simulink library "VIS_LIB"  (Simulink 8.6)
settings: Solver=ode45  StartTime=0.0  StopTime=10.0  RelTol=1e-3
undefined symbols (not defined in the file): AC, SIXOSEM_F_WD_AC_MASTER
libraries: cdsFilt x376, cdsEpicsOut x253, cdsEpicsIn x179, cdsTP x123, VIS_LIB x95, cdsMuxMatrix x91, cdsEpicsStringIn x75, cdsFiltCtrl x72, cdsFunctionCall x70, cdsRms x59, KAGRA_UTIL x25, STATE_BIO_MASTER x5
(part 19 of 38)

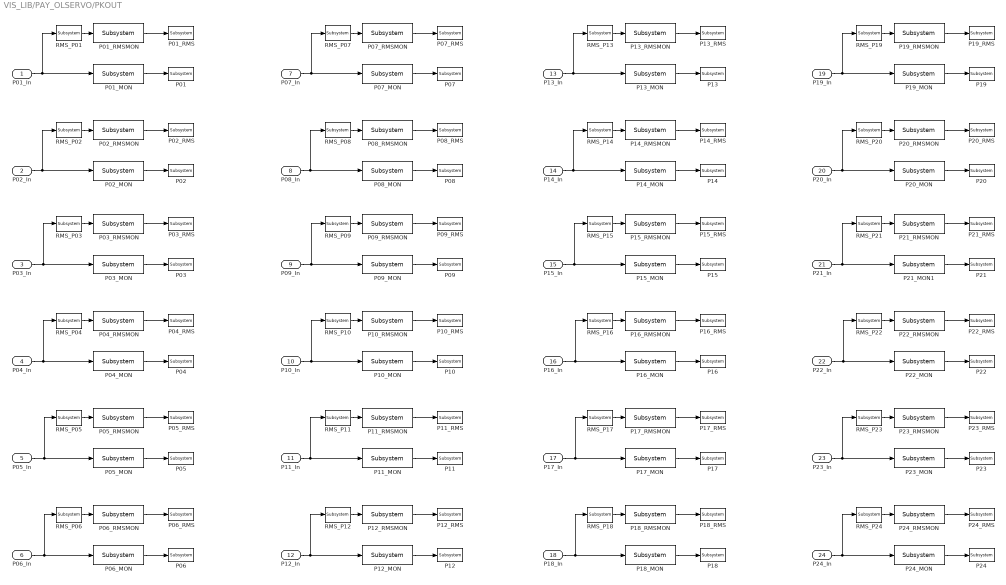
== system VIS_LIB/PAY_OLSERVO/PKOUT ==
  P01_In : Inport
  P02_In : Inport  Port=2
  P03_In : Inport  Port=3
  P04_In : Inport  Port=4
  P05_In : Inport  Port=5
  P06_In : Inport  Port=6
  P07_In : Inport  Port=7
  P08_In : Inport  Port=8
  P09_In : Inport  Port=9
  P10_In : Inport  Port=10
  P11_In : Inport  Port=11
  P12_In : Inport  Port=12
  P13_In : Inport  Port=13
  P14_In : Inport  Port=14
  P15_In : Inport  Port=15
  P16_In : Inport  Port=16
  P17_In : Inport  Port=17
  P18_In : Inport  Port=18
  P19_In : Inport  Port=19
  P20_In : Inport  Port=20
  P21_In : Inport  Port=21
  P22_In : Inport  Port=22
  P23_In : Inport  Port=23
  P24_In : Inport  Port=24
  P01 : cdsTP/Subsystem  Tag=Test Point
      settings: AttributesFormatString=%<Tag>
  P01_MON : cdsEpicsOut/Subsystem  Tag=cdsEpicsOutput  Description=|
      | Purpose:                                          
      | Output a FE signal to an EPICS channel.           
      |                                                   
      | Operation:                                        
      | Takes input value and passes it to EPICS record.  
      |                                                   
      | Usage:                                            
      | Name the part with the desired EPICS rrecord name.
      settings: AttributesFormatString=%<Tag>
  P01_RMS : cdsTP/Subsystem  Tag=Test Point
      settings: AttributesFormatString=%<Tag>
  P01_RMSMON : cdsEpicsOut/Subsystem  Tag=cdsEpicsOutput  Description=|
      | Purpose:                                          
      | Output a FE signal to an EPICS channel.           
      |                                                   
      | Operation:                                        
      | Takes input value and passes it to EPICS record.  
      |                                                   
      | Usage:                                            
      | Name the part with the desired EPICS rrecord name.
      settings: AttributesFormatString=%<Tag>
  P02 : cdsTP/Subsystem  Tag=Test Point
      settings: AttributesFormatString=%<Tag>
  P02_MON : cdsEpicsOut/Subsystem  Tag=cdsEpicsOutput  Description=|
      | Purpose:                                          
      | Output a FE signal to an EPICS channel.           
      |                                                   
      | Operation:                                        
      | Takes input value and passes it to EPICS record.  
      |                                                   
      | Usage:                                            
      | Name the part with the desired EPICS rrecord name.
      settings: AttributesFormatString=%<Tag>
  P02_RMS : cdsTP/Subsystem  Tag=Test Point
      settings: AttributesFormatString=%<Tag>
  P02_RMSMON : cdsEpicsOut/Subsystem  Tag=cdsEpicsOutput  Description=|
      | Purpose:                                          
      | Output a FE signal to an EPICS channel.           
      |                                                   
      | Operation:                                        
      | Takes input value and passes it to EPICS record.  
      |                                                   
      | Usage:                                            
      | Name the part with the desired EPICS rrecord name.
      settings: AttributesFormatString=%<Tag>
  P03 : cdsTP/Subsystem  Tag=Test Point
      settings: AttributesFormatString=%<Tag>
  P03_MON : cdsEpicsOut/Subsystem  Tag=cdsEpicsOutput  Description=|
      | Purpose:                                          
      | Output a FE signal to an EPICS channel.           
      |                                                   
      | Operation:                                        
      | Takes input value and passes it to EPICS record.  
      |                                                   
      | Usage:                                            
      | Name the part with the desired EPICS rrecord name.
      settings: AttributesFormatString=%<Tag>
  P03_RMS : cdsTP/Subsystem  Tag=Test Point
      settings: AttributesFormatString=%<Tag>
  P03_RMSMON : cdsEpicsOut/Subsystem  Tag=cdsEpicsOutput  Description=|
      | Purpose:                                          
      | Output a FE signal to an EPICS channel.           
      |                                                   
      | Operation:                                        
      | Takes input value and passes it to EPICS record.  
      |                                                   
      | Usage:                                            
      | Name the part with the desired EPICS rrecord name.
      settings: AttributesFormatString=%<Tag>
  P04 : cdsTP/Subsystem  Tag=Test Point
      settings: AttributesFormatString=%<Tag>
  P04_MON : cdsEpicsOut/Subsystem  Tag=cdsEpicsOutput  Description=|
      | Purpose:                                          
      | Output a FE signal to an EPICS channel.           
      |                                                   
      | Operation:                                        
      | Takes input value and passes it to EPICS record.  
      |                                                   
      | Usage:                                            
      | Name the part with the desired EPICS rrecord name.
      settings: AttributesFormatString=%<Tag>
  P04_RMS : cdsTP/Subsystem  Tag=Test Point
      settings: AttributesFormatString=%<Tag>
  P04_RMSMON : cdsEpicsOut/Subsystem  Tag=cdsEpicsOutput  Description=|
      | Purpose:                                          
      | Output a FE signal to an EPICS channel.           
      |                                                   
      | Operation:                                        
      | Takes input value and passes it to EPICS record.  
      |                                                   
      | Usage:                                            
      | Name the part with the desired EPICS rrecord name.
      settings: AttributesFormatString=%<Tag>
  P05 : cdsTP/Subsystem  Tag=Test Point
      settings: AttributesFormatString=%<Tag>
  P05_MON : cdsEpicsOut/Subsystem  Tag=cdsEpicsOutput  Description=|
      | Purpose:                                          
      | Output a FE signal to an EPICS channel.           
      |                                                   
      | Operation:                                        
      | Takes input value and passes it to EPICS record.  
      |                                                   
      | Usage:                                            
      | Name the part with the desired EPICS rrecord name.
      settings: AttributesFormatString=%<Tag>
  P05_RMS : cdsTP/Subsystem  Tag=Test Point
      settings: AttributesFormatString=%<Tag>
  P05_RMSMON : cdsEpicsOut/Subsystem  Tag=cdsEpicsOutput  Description=|
      | Purpose:                                          
      | Output a FE signal to an EPICS channel.           
      |                                                   
      | Operation:                                        
      | Takes input value and passes it to EPICS record.  
      |                                                   
      | Usage:                                            
      | Name the part with the desired EPICS rrecord name.
      settings: AttributesFormatString=%<Tag>
  P06 : cdsTP/Subsystem  Tag=Test Point
      settings: AttributesFormatString=%<Tag>
  P06_MON : cdsEpicsOut/Subsystem  Tag=cdsEpicsOutput  Description=|
      | Purpose:                                          
      | Output a FE signal to an EPICS channel.           
      |                                                   
      | Operation:                                        
      | Takes input value and passes it to EPICS record.  
      |                                                   
      | Usage:                                            
      | Name the part with the desired EPICS rrecord name.
      settings: AttributesFormatString=%<Tag>
  P06_RMS : cdsTP/Subsystem  Tag=Test Point
      settings: AttributesFormatString=%<Tag>
  P06_RMSMON : cdsEpicsOut/Subsystem  Tag=cdsEpicsOutput  Description=|
      | Purpose:                                          
      | Output a FE signal to an EPICS channel.           
      |                                                   
      | Operation:                                        
      | Takes input value and passes it to EPICS record.  
      |                                                   
      | Usage:                                            
      | Name the part with the desired EPICS rrecord name.
      settings: AttributesFormatString=%<Tag>
  P07 : cdsTP/Subsystem  Tag=Test Point
      settings: AttributesFormatString=%<Tag>
  P07_MON : cdsEpicsOut/Subsystem  Tag=cdsEpicsOutput  Description=|
      | Purpose:                                          
      | Output a FE signal to an EPICS channel.           
      |                                                   
      | Operation:                                        
      | Takes input value and passes it to EPICS record.  
      |                                                   
      | Usage:                                            
      | Name the part with the desired EPICS rrecord name.
      settings: AttributesFormatString=%<Tag>
  P07_RMS : cdsTP/Subsystem  Tag=Test Point
      settings: AttributesFormatString=%<Tag>
  P07_RMSMON : cdsEpicsOut/Subsystem  Tag=cdsEpicsOutput  Description=|
      | Purpose:                                          
      | Output a FE signal to an EPICS channel.           
      |                                                   
      | Operation:                                        
      | Takes input value and passes it to EPICS record.  
      |                                                   
      | Usage:                                            
      | Name the part with the desired EPICS rrecord name.
      settings: AttributesFormatString=%<Tag>
  P08 : cdsTP/Subsystem  Tag=Test Point
      settings: AttributesFormatString=%<Tag>
  P08_MON : cdsEpicsOut/Subsystem  Tag=cdsEpicsOutput  Description=|
      | Purpose:                                          
      | Output a FE signal to an EPICS channel.           
      |                                                   
      | Operation:                                        
      | Takes input value and passes it to EPICS record.  
      |                                                   
      | Usage:                                            
      | Name the part with the desired EPICS rrecord name.
      settings: AttributesFormatString=%<Tag>
  P08_RMS : cdsTP/Subsystem  Tag=Test Point
      settings: AttributesFormatString=%<Tag>
  P08_RMSMON : cdsEpicsOut/Subsystem  Tag=cdsEpicsOutput  Description=|
      | Purpose:                                          
      | Output a FE signal to an EPICS channel.           
      |                                                   
      | Operation:                                        
      | Takes input value and passes it to EPICS record.  
      |                                                   
      | Usage:                                            
      | Name the part with the desired EPICS rrecord name.
      settings: AttributesFormatString=%<Tag>
  P09 : cdsTP/Subsystem  Tag=Test Point
      settings: AttributesFormatString=%<Tag>
  P09_MON : cdsEpicsOut/Subsystem  Tag=cdsEpicsOutput  Description=|
      | Purpose:                                          
      | Output a FE signal to an EPICS channel.           
      |                                                   
      | Operation:                                        
      | Takes input value and passes it to EPICS record.  
      |                                                   
      | Usage:                                            
      | Name the part with the desired EPICS rrecord name.
      settings: AttributesFormatString=%<Tag>
  P09_RMS : cdsTP/Subsystem  Tag=Test Point
      settings: AttributesFormatString=%<Tag>
  P09_RMSMON : cdsEpicsOut/Subsystem  Tag=cdsEpicsOutput  Description=|
      | Purpose:                                          
      | Output a FE signal to an EPICS channel.           
      |                                                   
      | Operation:                                        
      | Takes input value and passes it to EPICS record.  
      |                                                   
      | Usage:                                            
      | Name the part with the desired EPICS rrecord name.
      settings: AttributesFormatString=%<Tag>
  P{10..24} (15 alike) : cdsTP/Subsystem  Tag=Test Point
      settings: AttributesFormatString=%<Tag>
  P10_MON : cdsEpicsOut/Subsystem  Tag=cdsEpicsOutput  Description=|
      | Purpose:                                          
      | Output a FE signal to an EPICS channel.           
      |                                                   
      | Operation:                                        
      | Takes input value and passes it to EPICS record.  
      |                                                   
      | Usage:                                            
      | Name the part with the desired EPICS rrecord name.
      settings: AttributesFormatString=%<Tag>
  P10_RMS : cdsTP/Subsystem  Tag=Test Point
      settings: AttributesFormatString=%<Tag>
  P10_RMSMON : cdsEpicsOut/Subsystem  Tag=cdsEpicsOutput  Description=|
      | Purpose:                                          
      | Output a FE signal to an EPICS channel.           
      |                                                   
      | Operation:                                        
      | Takes input value and passes it to EPICS record.  
      |                                                   
      | Usage:                                            
      | Name the part with the desired EPICS rrecord name.
      settings: AttributesFormatString=%<Tag>
  P11_MON : cdsEpicsOut/Subsystem  Tag=cdsEpicsOutput  Description=|
      | Purpose:                                          
      | Output a FE signal to an EPICS channel.           
      |                                                   
      | Operation:                                        
      | Takes input value and passes it to EPICS record.  
      |                                                   
      | Usage:                                            
      | Name the part with the desired EPICS rrecord name.
      settings: AttributesFormatString=%<Tag>
  P11_RMS : cdsTP/Subsystem  Tag=Test Point
      settings: AttributesFormatString=%<Tag>
  P11_RMSMON : cdsEpicsOut/Subsystem  Tag=cdsEpicsOutput  Description=|
      | Purpose:                                          
      | Output a FE signal to an EPICS channel.           
      |                                                   
      | Operation:                                        
      | Takes input value and passes it to EPICS record.  
      |                                                   
      | Usage:                                            
      | Name the part with the desired EPICS rrecord name.
      settings: AttributesFormatString=%<Tag>
  P12_MON : cdsEpicsOut/Subsystem  Tag=cdsEpicsOutput  Description=|
      | Purpose:                                          
      | Output a FE signal to an EPICS channel.           
      |                                                   
      | Operation:                                        
      | Takes input value and passes it to EPICS record.  
      |                                                   
      | Usage:                                            
      | Name the part with the desired EPICS rrecord name.
      settings: AttributesFormatString=%<Tag>
  P12_RMS : cdsTP/Subsystem  Tag=Test Point
      settings: AttributesFormatString=%<Tag>
  P12_RMSMON : cdsEpicsOut/Subsystem  Tag=cdsEpicsOutput  Description=|
      | Purpose:                                          
      | Output a FE signal to an EPICS channel.           
      |                                                   
      | Operation:                                        
      | Takes input value and passes it to EPICS record.  
      |                                                   
      | Usage:                                            
      | Name the part with the desired EPICS rrecord name.
      settings: AttributesFormatString=%<Tag>
  P13_MON : cdsEpicsOut/Subsystem  Tag=cdsEpicsOutput  Description=|
      | Purpose:                                          
      | Output a FE signal to an EPICS channel.           
      |                                                   
      | Operation:                                        
      | Takes input value and passes it to EPICS record.  
      |                                                   
      | Usage:                                            
      | Name the part with the desired EPICS rrecord name.
      settings: AttributesFormatString=%<Tag>
  P13_RMS : cdsTP/Subsystem  Tag=Test Point
      settings: AttributesFormatString=%<Tag>
  P13_RMSMON : cdsEpicsOut/Subsystem  Tag=cdsEpicsOutput  Description=|
      | Purpose:                                          
      | Output a FE signal to an EPICS channel.           
      |                                                   
      | Operation:                                        
      | Takes input value and passes it to EPICS record.  
      |                                                   
      | Usage:                                            
      | Name the part with the desired EPICS rrecord name.
      settings: AttributesFormatString=%<Tag>
  P14_MON : cdsEpicsOut/Subsystem  Tag=cdsEpicsOutput  Description=|
      | Purpose:                                          
      | Output a FE signal to an EPICS channel.           
      |                                                   
      | Operation:                                        
      | Takes input value and passes it to EPICS record.  
      |                                                   
      | Usage:                                            
      | Name the part with the desired EPICS rrecord name.
      settings: AttributesFormatString=%<Tag>
  P14_RMS : cdsTP/Subsystem  Tag=Test Point
      settings: AttributesFormatString=%<Tag>
  P14_RMSMON : cdsEpicsOut/Subsystem  Tag=cdsEpicsOutput  Description=|
      | Purpose:                                          
      | Output a FE signal to an EPICS channel.           
      |                                                   
      | Operation:                                        
      | Takes input value and passes it to EPICS record.  
      |                                                   
      | Usage:                                            
      | Name the part with the desired EPICS rrecord name.
      settings: AttributesFormatString=%<Tag>
  P15_MON : cdsEpicsOut/Subsystem  Tag=cdsEpicsOutput  Description=|
      | Purpose:                                          
      | Output a FE signal to an EPICS channel.           
      |                                                   
      | Operation:                                        
      | Takes input value and passes it to EPICS record.  
      |                                                   
      | Usage:                                            
      | Name the part with the desired EPICS rrecord name.
      settings: AttributesFormatString=%<Tag>
  P15_RMS : cdsTP/Subsystem  Tag=Test Point
      settings: AttributesFormatString=%<Tag>
  P15_RMSMON : cdsEpicsOut/Subsystem  Tag=cdsEpicsOutput  Description=|
      | Purpose:                                          
      | Output a FE signal to an EPICS channel.           
      |                                                   
      | Operation:                                        
      | Takes input value and passes it to EPICS record.  
      |                                                   
      | Usage:                                            
      | Name the part with the desired EPICS rrecord name.
      settings: AttributesFormatString=%<Tag>
  P16_MON : cdsEpicsOut/Subsystem  Tag=cdsEpicsOutput  Description=|
      | Purpose:                                          
      | Output a FE signal to an EPICS channel.           
      |                                                   
      | Operation:                                        
      | Takes input value and passes it to EPICS record.  
      |                                                   
      | Usage:                                            
      | Name the part with the desired EPICS rrecord name.
      settings: AttributesFormatString=%<Tag>
  P16_RMS : cdsTP/Subsystem  Tag=Test Point
      settings: AttributesFormatString=%<Tag>
  P16_RMSMON : cdsEpicsOut/Subsystem  Tag=cdsEpicsOutput  Description=|
      | Purpose:                                          
      | Output a FE signal to an EPICS channel.           
      |                                                   
      | Operation:                                        
      | Takes input value and passes it to EPICS record.  
      |                                                   
      | Usage:                                            
      | Name the part with the desired EPICS rrecord name.
      settings: AttributesFormatString=%<Tag>
  P17_MON : cdsEpicsOut/Subsystem  Tag=cdsEpicsOutput  Description=|
      | Purpose:                                          
      | Output a FE signal to an EPICS channel.           
      |                                                   
      | Operation:                                        
      | Takes input value and passes it to EPICS record.  
      |                                                   
      | Usage:                                            
      | Name the part with the desired EPICS rrecord name.
      settings: AttributesFormatString=%<Tag>
  P17_RMS : cdsTP/Subsystem  Tag=Test Point
      settings: AttributesFormatString=%<Tag>
  P17_RMSMON : cdsEpicsOut/Subsystem  Tag=cdsEpicsOutput  Description=|
      | Purpose:                                          
      | Output a FE signal to an EPICS channel.           
      |                                                   
      | Operation:                                        
      | Takes input value and passes it to EPICS record.  
      |                                                   
      | Usage:                                            
      | Name the part with the desired EPICS rrecord name.
      settings: AttributesFormatString=%<Tag>
  P18_MON : cdsEpicsOut/Subsystem  Tag=cdsEpicsOutput  Description=|
      | Purpose:                                          
      | Output a FE signal to an EPICS channel.           
      |                                                   
      | Operation:                                        
      | Takes input value and passes it to EPICS record.  
      |                                                   
      | Usage:                                            
      | Name the part with the desired EPICS rrecord name.
      settings: AttributesFormatString=%<Tag>
  P18_RMS : cdsTP/Subsystem  Tag=Test Point
      settings: AttributesFormatString=%<Tag>
  P18_RMSMON : cdsEpicsOut/Subsystem  Tag=cdsEpicsOutput  Description=|
      | Purpose:                                          
      | Output a FE signal to an EPICS channel.           
      |                                                   
      | Operation:                                        
      | Takes input value and passes it to EPICS record.  
      |                                                   
      | Usage:                                            
      | Name the part with the desired EPICS rrecord name.
      settings: AttributesFormatString=%<Tag>
  P19_MON : cdsEpicsOut/Subsystem  Tag=cdsEpicsOutput  Description=|
      | Purpose:                                          
      | Output a FE signal to an EPICS channel.           
      |                                                   
      | Operation:                                        
      | Takes input value and passes it to EPICS record.  
      |                                                   
      | Usage:                                            
      | Name the part with the desired EPICS rrecord name.
      settings: AttributesFormatString=%<Tag>
  P19_RMS : cdsTP/Subsystem  Tag=Test Point
      settings: AttributesFormatString=%<Tag>
  P19_RMSMON : cdsEpicsOut/Subsystem  Tag=cdsEpicsOutput  Description=|
      | Purpose:                                          
      | Output a FE signal to an EPICS channel.           
      |                                                   
      | Operation:                                        
      | Takes input value and passes it to EPICS record.  
      |                                                   
      | Usage:                                            
      | Name the part with the desired EPICS rrecord name.
      settings: AttributesFormatString=%<Tag>
  P20_MON : cdsEpicsOut/Subsystem  Tag=cdsEpicsOutput  Description=|
      | Purpose:                                          
      | Output a FE signal to an EPICS channel.           
      |                                                   
      | Operation:                                        
      | Takes input value and passes it to EPICS record.  
      |                                                   
      | Usage:                                            
      | Name the part with the desired EPICS rrecord name.
      settings: AttributesFormatString=%<Tag>
  P20_RMS : cdsTP/Subsystem  Tag=Test Point
      settings: AttributesFormatString=%<Tag>
  P20_RMSMON : cdsEpicsOut/Subsystem  Tag=cdsEpicsOutput  Description=|
      | Purpose:                                          
      | Output a FE signal to an EPICS channel.           
      |                                                   
      | Operation:                                        
      | Takes input value and passes it to EPICS record.  
      |                                                   
      | Usage:                                            
      | Name the part with the desired EPICS rrecord name.
      settings: AttributesFormatString=%<Tag>
  P21_MON1 : cdsEpicsOut/Subsystem  Tag=cdsEpicsOutput  Description=|
      | Purpose:                                          
      | Output a FE signal to an EPICS channel.           
      |                                                   
      | Operation:                                        
      | Takes input value and passes it to EPICS record.  
      |                                                   
      | Usage:                                            
      | Name the part with the desired EPICS rrecord name.
      settings: AttributesFormatString=%<Tag>
  P21_RMS : cdsTP/Subsystem  Tag=Test Point
      settings: AttributesFormatString=%<Tag>
  P21_RMSMON : cdsEpicsOut/Subsystem  Tag=cdsEpicsOutput  Description=|
      | Purpose:                                          
      | Output a FE signal to an EPICS channel.           
      |                                                   
      | Operation:                                        
      | Takes input value and passes it to EPICS record.  
      |                                                   
      | Usage:                                            
      | Name the part with the desired EPICS rrecord name.
      settings: AttributesFormatString=%<Tag>
  P22_MON : cdsEpicsOut/Subsystem  Tag=cdsEpicsOutput  Description=|
      | Purpose:                                          
      | Output a FE signal to an EPICS channel.           
      |                                                   
      | Operation:                                        
      | Takes input value and passes it to EPICS record.  
      |                                                   
      | Usage:                                            
      | Name the part with the desired EPICS rrecord name.
      settings: AttributesFormatString=%<Tag>
  P22_RMS : cdsTP/Subsystem  Tag=Test Point
      settings: AttributesFormatString=%<Tag>
  P22_RMSMON : cdsEpicsOut/Subsystem  Tag=cdsEpicsOutput  Description=|
      | Purpose:                                          
      | Output a FE signal to an EPICS channel.           
      |                                                   
      | Operation:                                        
      | Takes input value and passes it to EPICS record.  
      |                                                   
      | Usage:                                            
      | Name the part with the desired EPICS rrecord name.
      settings: AttributesFormatString=%<Tag>
  P23_MON : cdsEpicsOut/Subsystem  Tag=cdsEpicsOutput  Description=|
      | Purpose:                                          
      | Output a FE signal to an EPICS channel.           
      |                                                   
      | Operation:                                        
      | Takes input value and passes it to EPICS record.  
      |                                                   
      | Usage:                                            
      | Name the part with the desired EPICS rrecord name.
      settings: AttributesFormatString=%<Tag>
  P23_RMS : cdsTP/Subsystem  Tag=Test Point
      settings: AttributesFormatString=%<Tag>
  P23_RMSMON : cdsEpicsOut/Subsystem  Tag=cdsEpicsOutput  Description=|
      | Purpose:                                          
      | Output a FE signal to an EPICS channel.           
      |                                                   
      | Operation:                                        
      | Takes input value and passes it to EPICS record.  
      |                                                   
      | Usage:                                            
      | Name the part with the desired EPICS rrecord name.
      settings: AttributesFormatString=%<Tag>
  P24_MON : cdsEpicsOut/Subsystem  Tag=cdsEpicsOutput  Description=|
      | Purpose:                                          
      | Output a FE signal to an EPICS channel.           
      |                                                   
      | Operation:                                        
      | Takes input value and passes it to EPICS record.  
      |                                                   
      | Usage:                                            
      | Name the part with the desired EPICS rrecord name.
      settings: AttributesFormatString=%<Tag>
  P24_RMS : cdsTP/Subsystem  Tag=Test Point
      settings: AttributesFormatString=%<Tag>
  P24_RMSMON : cdsEpicsOut/Subsystem  Tag=cdsEpicsOutput  Description=|
      | Purpose:                                          
      | Output a FE signal to an EPICS channel.           
      |                                                   
      | Operation:                                        
      | Takes input value and passes it to EPICS record.  
      |                                                   
      | Usage:                                            
      | Name the part with the desired EPICS rrecord name.
      settings: AttributesFormatString=%<Tag>
  RMS_P01 : cdsRms/Subsystem  Tag=cdsRms  Description=|
      | Purpose:
      | Calculate an RMS based on the input signal.
      settings: AttributesFormatString=%<Tag>
  RMS_P02 : cdsRms/Subsystem  Tag=cdsRms  Description=|
      | Purpose:
      | Calculate an RMS based on the input signal.
      settings: AttributesFormatString=%<Tag>
  RMS_P03 : cdsRms/Subsystem  Tag=cdsRms  Description=|
      | Purpose:
      | Calculate an RMS based on the input signal.
      settings: AttributesFormatString=%<Tag>
  RMS_P04 : cdsRms/Subsystem  Tag=cdsRms  Description=|
      | Purpose:
      | Calculate an RMS based on the input signal.
      settings: AttributesFormatString=%<Tag>
  RMS_P05 : cdsRms/Subsystem  Tag=cdsRms  Description=|
      | Purpose:
      | Calculate an RMS based on the input signal.
      settings: AttributesFormatString=%<Tag>
  RMS_P06 : cdsRms/Subsystem  Tag=cdsRms  Description=|
      | Purpose:
      | Calculate an RMS based on the input signal.
      settings: AttributesFormatString=%<Tag>
  RMS_P07 : cdsRms/Subsystem  Tag=cdsRms  Description=|
      | Purpose:
      | Calculate an RMS based on the input signal.
      settings: AttributesFormatString=%<Tag>
  RMS_P08 : cdsRms/Subsystem  Tag=cdsRms  Description=|
      | Purpose:
      | Calculate an RMS based on the input signal.
      settings: AttributesFormatString=%<Tag>
  RMS_P09 : cdsRms/Subsystem  Tag=cdsRms  Description=|
      | Purpose:
      | Calculate an RMS based on the input signal.
      settings: AttributesFormatString=%<Tag>
  RMS_P{10..24} (15 alike) : cdsRms/Subsystem  Tag=cdsRms  Description=|
      | Purpose:
      | Calculate an RMS based on the input signal.
      settings: AttributesFormatString=%<Tag>
  wires:
  P03_In/1 -> RMS_P03/1, P03_MON/1
  P03_MON/1 -> P03/1
  P02_In/1 -> RMS_P02/1, P02_MON/1
  P02_MON/1 -> P02/1
  P01_In/1 -> RMS_P01/1, P01_MON/1
  P01_MON/1 -> P01/1
  P06_In/1 -> RMS_P06/1, P06_MON/1
  P06_MON/1 -> P06/1
  P05_In/1 -> RMS_P05/1, P05_MON/1
  P05_MON/1 -> P05/1
  P04_In/1 -> RMS_P04/1, P04_MON/1
  P04_MON/1 -> P04/1
  P09_MON/1 -> P09/1
  P08_MON/1 -> P08/1
  P07_MON/1 -> P07/1
  P12_MON/1 -> P12/1
  P11_MON/1 -> P11/1
  P10_MON/1 -> P10/1
  P01_RMSMON/1 -> P01_RMS/1
  RMS_P01/1 -> P01_RMSMON/1
  P02_RMSMON/1 -> P02_RMS/1
  RMS_P02/1 -> P02_RMSMON/1
  P03_RMSMON/1 -> P03_RMS/1
  RMS_P03/1 -> P03_RMSMON/1
  P04_RMSMON/1 -> P04_RMS/1
  RMS_P04/1 -> P04_RMSMON/1
  P05_RMSMON/1 -> P05_RMS/1
  RMS_P05/1 -> P05_RMSMON/1
  P06_RMSMON/1 -> P06_RMS/1
  RMS_P06/1 -> P06_RMSMON/1
  P07_In/1 -> RMS_P07/1, P07_MON/1
  P07_RMSMON/1 -> P07_RMS/1
  RMS_P07/1 -> P07_RMSMON/1
  P08_In/1 -> RMS_P08/1, P08_MON/1
  P08_RMSMON/1 -> P08_RMS/1
  RMS_P08/1 -> P08_RMSMON/1
  P09_In/1 -> RMS_P09/1, P09_MON/1
  P09_RMSMON/1 -> P09_RMS/1
  RMS_P09/1 -> P09_RMSMON/1
  P10_In/1 -> RMS_P10/1, P10_MON/1
  P10_RMSMON/1 -> P10_RMS/1
  RMS_P10/1 -> P10_RMSMON/1
  P11_In/1 -> RMS_P11/1, P11_MON/1
  P11_RMSMON/1 -> P11_RMS/1
  RMS_P11/1 -> P11_RMSMON/1
  P12_In/1 -> RMS_P12/1, P12_MON/1
  P12_RMSMON/1 -> P12_RMS/1
  RMS_P12/1 -> P12_RMSMON/1
  P15_In/1 -> RMS_P15/1, P15_MON/1
  P15_MON/1 -> P15/1
  P14_In/1 -> RMS_P14/1, P14_MON/1
  P14_MON/1 -> P14/1
  P13_In/1 -> RMS_P13/1, P13_MON/1
  P13_MON/1 -> P13/1
  P18_In/1 -> RMS_P18/1, P18_MON/1
  P18_MON/1 -> P18/1
  P17_In/1 -> RMS_P17/1, P17_MON/1
  P17_MON/1 -> P17/1
  P16_In/1 -> RMS_P16/1, P16_MON/1
  P16_MON/1 -> P16/1
  P21_MON1/1 -> P21/1
  P20_MON/1 -> P20/1
  P19_MON/1 -> P19/1
  P24_MON/1 -> P24/1
  P23_MON/1 -> P23/1
  P22_MON/1 -> P22/1
  P13_RMSMON/1 -> P13_RMS/1
  RMS_P13/1 -> P13_RMSMON/1
  P14_RMSMON/1 -> P14_RMS/1
  RMS_P14/1 -> P14_RMSMON/1
  P15_RMSMON/1 -> P15_RMS/1
  RMS_P15/1 -> P15_RMSMON/1
  P16_RMSMON/1 -> P16_RMS/1
  RMS_P16/1 -> P16_RMSMON/1
  P17_RMSMON/1 -> P17_RMS/1
  RMS_P17/1 -> P17_RMSMON/1
  P18_RMSMON/1 -> P18_RMS/1
  RMS_P18/1 -> P18_RMSMON/1
  P19_In/1 -> RMS_P19/1, P19_MON/1
  P19_RMSMON/1 -> P19_RMS/1
  RMS_P19/1 -> P19_RMSMON/1
  P20_In/1 -> RMS_P20/1, P20_MON/1
  P20_RMSMON/1 -> P20_RMS/1
  RMS_P20/1 -> P20_RMSMON/1
  P21_In/1 -> RMS_P21/1, P21_MON1/1
  P21_RMSMON/1 -> P21_RMS/1
  RMS_P21/1 -> P21_RMSMON/1
  P22_In/1 -> RMS_P22/1, P22_MON/1
  P22_RMSMON/1 -> P22_RMS/1
  RMS_P22/1 -> P22_RMSMON/1
  P23_In/1 -> RMS_P23/1, P23_MON/1
  P23_RMSMON/1 -> P23_RMS/1
  RMS_P23/1 -> P23_RMSMON/1
  P24_In/1 -> RMS_P24/1, P24_MON/1
  P24_RMSMON/1 -> P24_RMS/1
  RMS_P24/1 -> P24_RMSMON/1
